simulink subsystem "LVSS"  (R2025b)
settings: Solver=VariableStepAuto  StartTime=0.0  StopTime=10.0  RelTol=1e-3
PreLoadFcn:
  | HIB_Current = 18;
libraries: simulink x1
settings Model: Creator=matat  LastModifiedBy=matat
settings RTWCC: GPUComputeCapability=3.5

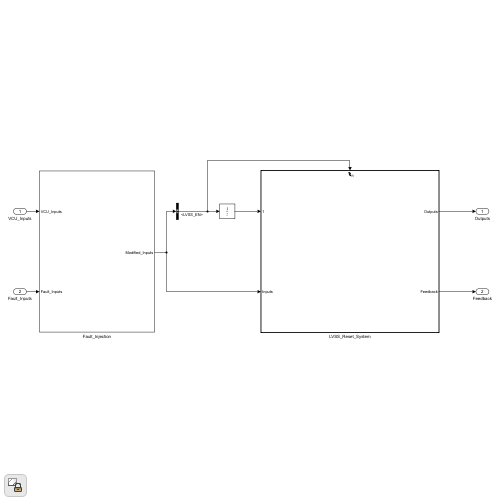
[thumbnail: Simulink's stored preview of the top-level diagram]
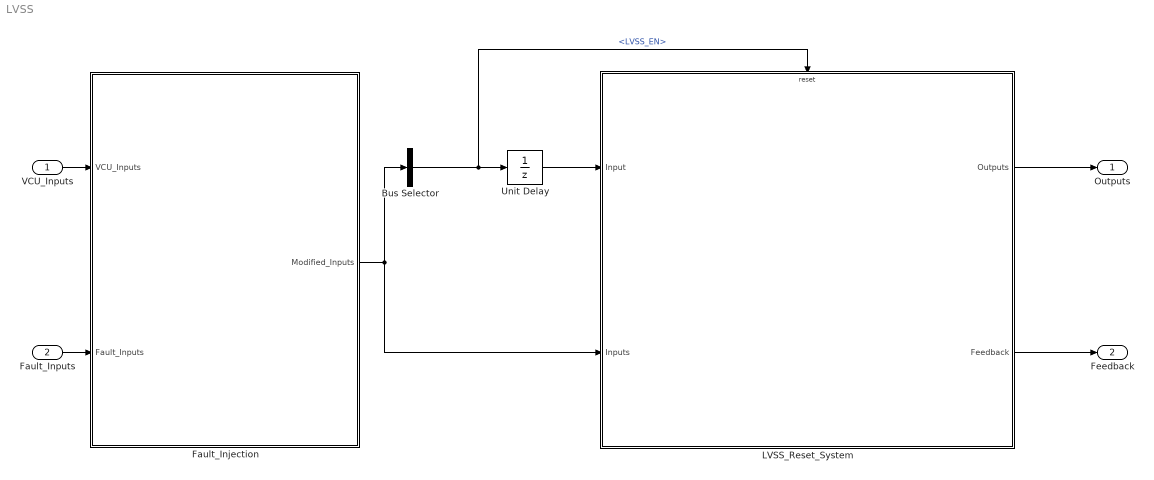
== system LVSS ==
  VCU_Inputs : Inport
  Fault_Inputs : Inport  Port=2
  Bus Selector : BusSelector  OutputSignals=LVSS_EN
  Fault_Injection : Subsystem
  LVSS_Reset_System : Subsystem  TreatAsAtomicUnit=on
  Unit Delay : UnitDelay  SampleTime=-1  HasFrameUpgradeWarning=on
  Outputs : Outport
  Feedback : Outport  Port=2
  wires:
  VCU_Inputs/1 -> Fault_Injection/1(VCU_Inputs)
  Fault_Inputs/1 -> Fault_Injection/2(Fault_Inputs)
  LVSS_Reset_System/1(Outputs) -> Outputs/1
  LVSS_Reset_System/2(Feedback) -> Feedback/1
  Fault_Injection/1(Modified_Inputs) -> Bus Selector/1, LVSS_Reset_System/2(Inputs)
  Unit Delay/1 -> LVSS_Reset_System/1(Input)
  Bus Selector/1 -> Unit Delay/1, LVSS_Reset_System/Reset  "<LVSS_EN>"

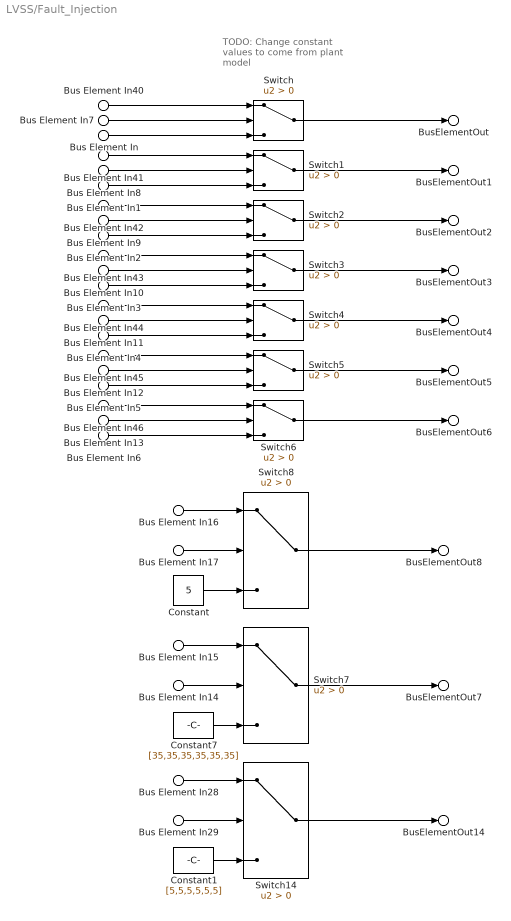
== system LVSS/Fault_Injection ==
  note: TODO: Change constant values to come from plant model
  Bus Element In6 : Inport  PortName=VCU_Inputs  Element=LVSS_Outputs.Batt_12V_EN
  Bus Element In1 : Inport  PortName=VCU_Inputs  Element=LVSS_Outputs.TMS_EN
  Bus Element In2 : Inport  PortName=VCU_Inputs  Element=LVSS_Outputs.GUB_EN
  Bus Element In3 : Inport  PortName=VCU_Inputs  Element=LVSS_Outputs.HIB_EN
  Bus Element In4 : Inport  PortName=VCU_Inputs  Element=LVSS_Outputs.HUDL_EN
  Bus Element In5 : Inport  PortName=VCU_Inputs  Element=LVSS_Outputs.Acc_EN
  Bus Element In : Inport  PortName=VCU_Inputs  Element=LVSS_Outputs.LVSS_EN
  Bus Element In7 : Inport  Port=2  PortName=Fault_Inputs  Element=Override_LVSS_EN
  Bus Element In8 : Inport  Port=2  PortName=Fault_Inputs  Element=Override_TMS_EN
  Bus Element In9 : Inport  Port=2  PortName=Fault_Inputs  Element=Override_GUB_EN
  Bus Element In10 : Inport  Port=2  PortName=Fault_Inputs  Element=Override_HIB_EN
  Bus Element In11 : Inport  Port=2  PortName=Fault_Inputs  Element=Override_HUDL_EN
  Bus Element In12 : Inport  Port=2  PortName=Fault_Inputs  Element=Override_Acc_EN
  Bus Element In13 : Inport  Port=2  PortName=Fault_Inputs  Element=Override_Batt_12V_EN
  Bus Element In16 : Inport  Port=2  PortName=Fault_Inputs  Element=Vicor_Current
  Bus Element In17 : Inport  Port=2  PortName=Fault_Inputs  Element=Override_Vicor_Current
  Bus Element In15 : Inport  Port=2  PortName=Fault_Inputs  Element=LVSS_Temps
  Bus Element In14 : Inport  Port=2  PortName=Fault_Inputs  Element=Override_LVSS_Temps
  Bus Element In28 : Inport  Port=2  PortName=Fault_Inputs  Element=LVSS_Currents
  Bus Element In29 : Inport  Port=2  PortName=Fault_Inputs  Element=Override_LVSS_Currents
  Bus Element In40 : Inport  Port=2  PortName=Fault_Inputs  Element=LVSS_EN
  Bus Element In41 : Inport  Port=2  PortName=Fault_Inputs  Element=TMS_EN
  Bus Element In42 : Inport  Port=2  PortName=Fault_Inputs  Element=GUB_EN
  Bus Element In43 : Inport  Port=2  PortName=Fault_Inputs  Element=HIB_EN
  Bus Element In44 : Inport  Port=2  PortName=Fault_Inputs  Element=HUDL_EN
  Bus Element In45 : Inport  Port=2  PortName=Fault_Inputs  Element=Acc_EN
  Bus Element In46 : Inport  Port=2  PortName=Fault_Inputs  Element=Batt_12V_EN
  Constant : Constant  Value=5  OutDataTypeStr=int16
  Constant1 : Constant  Value=[5,5,5,5,5,5]
  Constant7 : Constant  Value=[35,35,35,35,35,35]  OutDataTypeStr=int16
  Switch : Switch  Criteria=u2 > Threshold  OutDataTypeStr=boolean  SaturateOnIntegerOverflow=off  InputSameDT=off
  Switch{1..6,8,14} (8 alike) : Switch  Criteria=u2 > Threshold  SaturateOnIntegerOverflow=off  InputSameDT=off
  Switch7 : Switch  Criteria=u2 > Threshold  OutDataTypeStr=int16  SaturateOnIntegerOverflow=off  InputSameDT=off
  BusElementOut : Outport  PortName=Modified_Inputs  Element=LVSS_EN
  BusElementOut1 : Outport  PortName=Modified_Inputs  Element=TMS_EN
  BusElementOut2 : Outport  PortName=Modified_Inputs  Element=GUB_EN
  BusElementOut3 : Outport  PortName=Modified_Inputs  Element=HIB_EN
  BusElementOut4 : Outport  PortName=Modified_Inputs  Element=HUDL_EN
  BusElementOut5 : Outport  PortName=Modified_Inputs  Element=Acc_EN
  BusElementOut6 : Outport  PortName=Modified_Inputs  Element=Batt_12V_EN
  BusElementOut8 : Outport  PortName=Modified_Inputs  Element=Vicor_Current
  BusElementOut7 : Outport  PortName=Modified_Inputs  Element=LVSS_Temps
  BusElementOut14 : Outport  PortName=Modified_Inputs  Element=LVSS_Currents
  wires:
  Switch/1 -> BusElementOut/1
  Switch1/1 -> BusElementOut1/1
  Switch2/1 -> BusElementOut2/1
  Switch3/1 -> BusElementOut3/1
  Switch4/1 -> BusElementOut4/1
  Switch5/1 -> BusElementOut5/1
  Switch6/1 -> BusElementOut6/1
  Bus Element In/1 -> Switch/3
  Bus Element In1/1 -> Switch1/3
  Bus Element In2/1 -> Switch2/3
  Bus Element In3/1 -> Switch3/3
  Bus Element In4/1 -> Switch4/3
  Bus Element In5/1 -> Switch5/3
  Bus Element In6/1 -> Switch6/3
  Bus Element In40/1 -> Switch/1
  Bus Element In41/1 -> Switch1/1
  Bus Element In42/1 -> Switch2/1
  Bus Element In43/1 -> Switch3/1
  Bus Element In44/1 -> Switch4/1
  Bus Element In45/1 -> Switch5/1
  Bus Element In46/1 -> Switch6/1
  Bus Element In7/1 -> Switch/2
  Bus Element In8/1 -> Switch1/2
  Bus Element In9/1 -> Switch2/2
  Bus Element In10/1 -> Switch3/2
  Bus Element In11/1 -> Switch4/2
  Bus Element In12/1 -> Switch5/2
  Bus Element In13/1 -> Switch6/2
  Bus Element In15/1 -> Switch7/1
  Bus Element In14/1 -> Switch7/2
  Constant7/1 -> Switch7/3
  Switch7/1 -> BusElementOut7/1
  Constant/1 -> Switch8/3
  Bus Element In16/1 -> Switch8/1
  Bus Element In17/1 -> Switch8/2
  Switch8/1 -> BusElementOut8/1
  Constant1/1 -> Switch14/3
  Bus Element In29/1 -> Switch14/2
  Switch14/1 -> BusElementOut14/1
  Bus Element In28/1 -> Switch14/1

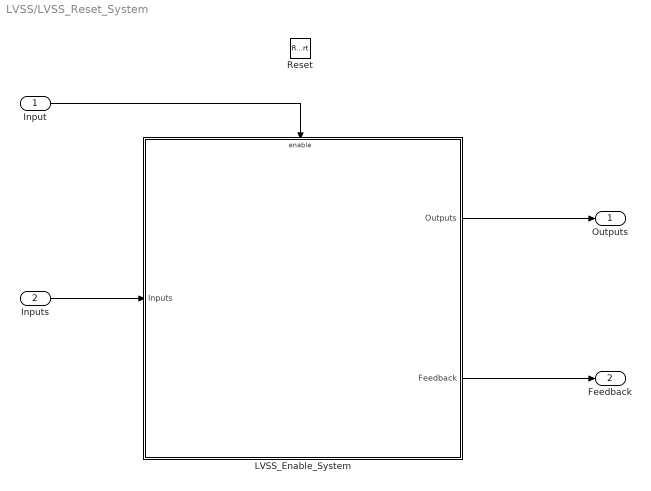
== system LVSS/LVSS_Reset_System ==
  Input : Inport
  Inputs : Inport  Port=2
  Reset : ResetPort  DisableCoverage=on  ResetTriggerType=falling
  "LVSS_Enable_System " : Subsystem  TreatAsAtomicUnit=on
  Outputs : Outport
  Feedback : Outport  Port=2
  wires:
  "LVSS_Enable_System "/1(Outputs) -> Outputs/1
  "LVSS_Enable_System "/2(Feedback) -> Feedback/1
  Inputs/1 -> "LVSS_Enable_System "/1(Inputs)
  Input/1 -> "LVSS_Enable_System "/Enable

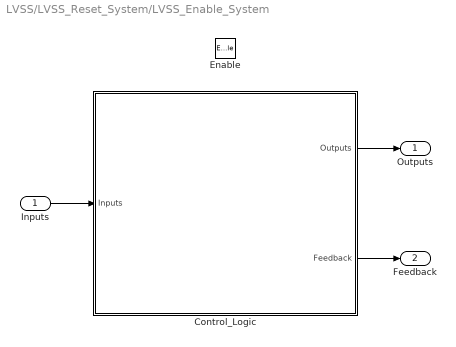
== system LVSS/LVSS_Reset_System/LVSS_Enable_System  ==
  Inputs : Inport
  Enable : EnablePort  StatesWhenEnabling=reset
  Control_Logic : Subsystem
  Outputs : Outport
  Feedback : Outport  Port=2
  wires:
  Control_Logic/2(Feedback) -> Feedback/1
  Control_Logic/1(Outputs) -> Outputs/1
  Inputs/1 -> Control_Logic/1(Inputs)

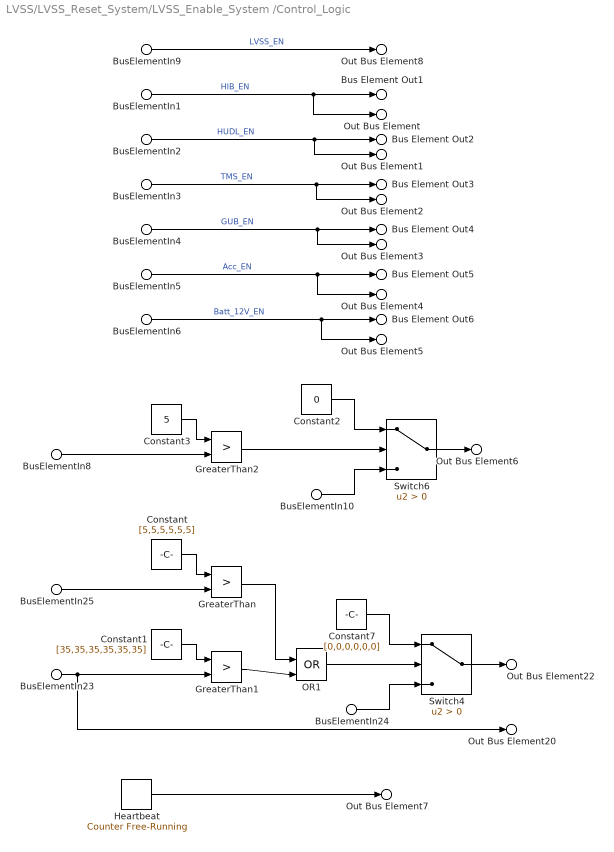
== system LVSS/LVSS_Reset_System/LVSS_Enable_System /Control_Logic ==
  BusElementIn9 : Inport  PortName=Inputs  Element=LVSS_EN
  BusElementIn1 : Inport  PortName=Inputs  Element=HIB_EN
  BusElementIn2 : Inport  PortName=Inputs  Element=HUDL_EN
  BusElementIn3 : Inport  PortName=Inputs  Element=TMS_EN
  BusElementIn4 : Inport  PortName=Inputs  Element=GUB_EN
  BusElementIn5 : Inport  PortName=Inputs  Element=Acc_EN
  BusElementIn6 : Inport  PortName=Inputs  Element=Batt_12V_EN
  BusElementIn23 : Inport  PortName=Inputs  Element=LVSS_Temps
  BusElementIn8 : Inport  PortName=Inputs  Element=Vicor_Current
  BusElementIn10 : Inport  PortName=Inputs  Element=Vicor_Current
  BusElementIn24 : Inport  PortName=Inputs  Element=LVSS_Currents
  BusElementIn25 : Inport  PortName=Inputs  Element=LVSS_Currents
  Constant : Constant  Value=[5,5,5,5,5,5]
  Constant1 : Constant  Value=[35,35,35,35,35,35]
  Constant2 : Constant  Value=0
  Constant3 : Constant  Value=5
  Constant7 : Constant  Value=[0,0,0,0,0,0]
  GreaterThan : RelationalOperator  Operator=>  OutDataTypeStr=boolean  RndMeth=Simplest  InputSameDT=off
  GreaterThan1 : RelationalOperator  Operator=>  OutDataTypeStr=boolean  RndMeth=Simplest  InputSameDT=off
  GreaterThan2 : RelationalOperator  Operator=>  OutDataTypeStr=boolean  RndMeth=Simplest  InputSameDT=off
  Heartbeat : simulink/Sources/Counter Free-Running  NumBits=32  tsamp=-1
  OR1 : Logic  Operator=OR  IconShape=distinctive  AllPortsSameDT=off  OutDataTypeStr=boolean
  Switch4 : Switch  Criteria=u2 > Threshold  SaturateOnIntegerOverflow=off  InputSameDT=off
  Switch6 : Switch  Criteria=u2 > Threshold  SaturateOnIntegerOverflow=off  InputSameDT=off
  Bus Element Out1 : Outport  PortName=Outputs  Element=HIB_Power
  Bus Element Out2 : Outport  PortName=Outputs  Element=HUDL_Power
  Bus Element Out3 : Outport  PortName=Outputs  Element=TMS_Power
  Bus Element Out4 : Outport  PortName=Outputs  Element=GUB_Power
  Bus Element Out5 : Outport  PortName=Outputs  Element=Acc_Power
  Bus Element Out6 : Outport  PortName=Outputs  Element=Batt_12V_Power
  Out Bus Element : Outport  Port=2  PortName=Feedback  Element=HIB_ON
  Out Bus Element1 : Outport  Port=2  PortName=Feedback  Element=HUDL_ON
  Out Bus Element2 : Outport  Port=2  PortName=Feedback  Element=TMS_ON
  Out Bus Element3 : Outport  Port=2  PortName=Feedback  Element=GUB_ON
  Out Bus Element4 : Outport  Port=2  PortName=Feedback  Element=Acc_ON
  Out Bus Element5 : Outport  Port=2  PortName=Feedback  Element=Batt_12V_ON
  Out Bus Element8 : Outport  Port=2  PortName=Feedback  Element=LVSS_ON
  Out Bus Element6 : Outport  Port=2  PortName=Feedback  Element=Vicor_Current
  Out Bus Element20 : Outport  Port=2  PortName=Feedback  Element=LVSS_Temps
  Out Bus Element22 : Outport  Port=2  PortName=Feedback  Element=LVSS_Currents
  Out Bus Element7 : Outport  Port=2  PortName=Feedback  Element=LVSS_Heartbeat
  wires:
  Constant3/1 -> GreaterThan2/1
  BusElementIn5/1 -> Out Bus Element4/1, Bus Element Out5/1  "Acc_EN"
  BusElementIn25/1 -> GreaterThan/2
  Constant7/1 -> Switch4/1
  GreaterThan1/1 -> OR1/2
  Constant1/1 -> GreaterThan1/1
  Switch4/1 -> Out Bus Element22/1
  BusElementIn4/1 -> Out Bus Element3/1, Bus Element Out4/1  "GUB_EN"
  Constant2/1 -> Switch6/1
  GreaterThan2/1 -> Switch6/2
  BusElementIn9/1 -> Out Bus Element8/1  "LVSS_EN"
  GreaterThan/1 -> OR1/1
  BusElementIn3/1 -> Out Bus Element2/1, Bus Element Out3/1  "TMS_EN"
  Switch6/1 -> Out Bus Element6/1
  BusElementIn6/1 -> Out Bus Element5/1, Bus Element Out6/1  "Batt_12V_EN"
  BusElementIn10/1 -> Switch6/3
  BusElementIn23/1 -> GreaterThan1/2, Out Bus Element20/1
  BusElementIn24/1 -> Switch4/3
  Constant/1 -> GreaterThan/1
  Heartbeat/1 -> Out Bus Element7/1
  BusElementIn8/1 -> GreaterThan2/2
  OR1/1 -> Switch4/2
  BusElementIn2/1 -> Out Bus Element1/1, Bus Element Out2/1  "HUDL_EN"
  BusElementIn1/1 -> Out Bus Element/1, Bus Element Out1/1  "HIB_EN"
